simulink model "lato_pc_def"  (Simulink 7.7)
settings: Solver=ode45  StartTime=0.0  StopTime=10.0  RelTol=1e-3
undefined symbols (not defined in the file): DiscIntNeverNeededParam
settings Model: Creator=valeria  LastModifiedBy=valeria

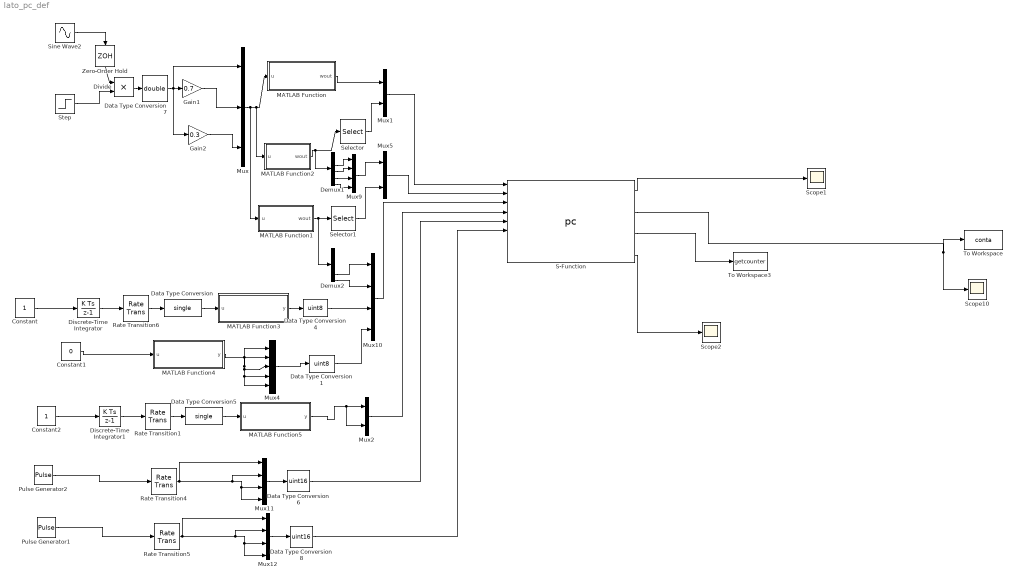
== system lato_pc_def ==
  Constant : Constant  OutDataTypeStr=single
  Constant1 : Constant  Value=0  OutDataTypeStr=single
  Constant2 : Constant  OutDataTypeStr=single
  Data Type Conversion : DataTypeConversion  OutDataTypeStr=single
  Data Type Conversion1 : DataTypeConversion  OutDataTypeStr=uint8
  Data Type Conversion4 : DataTypeConversion  OutDataTypeStr=uint8
  Data Type Conversion5 : DataTypeConversion  OutDataTypeStr=single
  Data Type Conversion6 : DataTypeConversion  OutDataTypeStr=uint16
  Data Type Conversion7 : DataTypeConversion  OutDataTypeStr=double
  Data Type Conversion8 : DataTypeConversion  OutDataTypeStr=uint16
  Demux1 : Demux  Outputs=6
  Demux2 : Demux  Outputs=6
  Discrete-Time Integrator : DiscreteIntegrator  gainval=100  SampleTime=-1  OutDataTypeStr=uint16  ICPrevOutput=DiscIntNeverNeededParam  ICPrevScaledInput=DiscIntNeverNeededParam
  Discrete-Time Integrator1 : DiscreteIntegrator  gainval=100  SampleTime=-1  OutDataTypeStr=uint16  ICPrevOutput=DiscIntNeverNeededParam  ICPrevScaledInput=DiscIntNeverNeededParam
  Divide : Product  Inputs=**
  Gain1 : Gain  Gain=0.7
  Gain2 : Gain  Gain=0.3
  MATLAB Function : Stateflow chart  TreatAsAtomicUnit=on
  MATLAB Function1 : Stateflow chart  TreatAsAtomicUnit=on
  MATLAB Function2 : Stateflow chart  TreatAsAtomicUnit=on
  MATLAB Function3 : Stateflow chart  TreatAsAtomicUnit=on
  MATLAB Function4 : Stateflow chart  TreatAsAtomicUnit=on
  MATLAB Function5 : Stateflow chart  TreatAsAtomicUnit=on
  Mux : Mux  Inputs=3
  Mux1 : Mux  Inputs=2
  Mux{9..12} (4 alike) : Mux
  Mux2 : Mux  Inputs=2
  Mux4 : Mux  Inputs=5
  Mux5 : Mux  Inputs=2
  Pulse Generator1 : DiscretePulseGenerator  PulseType=Time based  Period=10  PulseWidth=5
  Pulse Generator2 : DiscretePulseGenerator  PulseType=Time based  Period=10  PulseWidth=5
  Rate Transition1 : RateTransition
  Rate Transition4 : RateTransition  Deterministic=off
  Rate Transition5 : RateTransition  Deterministic=off
  Rate Transition6 : RateTransition
  S-Function : S-Function  FunctionName=pc  EnableBusSupport=off
  Scope1 : Scope
      settings: YMin=11628  YMax=12852  SaveName=ScopeData2
  Scope10 : Scope
  Scope2 : Scope
      settings: YMin=11628  YMax=12852
  Selector : Selector  InputPortWidth=6  IndexOptions=Index vector (dialog)  Indices=[1 2]  OutputSizes=1
  Selector1 : Selector  InputPortWidth=6  IndexOptions=Index vector (dialog)  Indices=[1 2 3 4]  OutputSizes=1
  Sine Wave2 : Sin  Amplitude=2500*pi/180  SampleTime=0
  Step : Step  SampleTime=0
  To Workspace : ToWorkspace  VariableName=conta  SampleTime=-1  SaveFormat=Structure
  To Workspace3 : ToWorkspace  VariableName=getcounter  SampleTime=-1  SaveFormat=Structure
  Zero-Order Hold : ZeroOrderHold  SampleTime=0.01
  wires:
  S-Function/1 -> Scope1/1
  S-Function/2 -> Scope10/1, To Workspace/1
  S-Function/3 -> To Workspace3/1
  Mux/1 -> MATLAB Function/1(u), MATLAB Function2/1(u), MATLAB Function1/1(u)
  Sine Wave2/1 -> Zero-Order Hold/1
  Data Type Conversion7/1 -> Gain1/1, Mux/1, Gain2/1
  Zero-Order Hold/1 -> Divide/1
  Step/1 -> Divide/2
  Divide/1 -> Data Type Conversion7/1
  Gain2/1 -> Mux/3
  Gain1/1 -> Mux/2
  MATLAB Function2/1(wout) -> Selector/1, Demux1/1
  MATLAB Function/1(wout) -> Mux1/1
  Selector/1 -> Mux1/2
  Mux1/1 -> S-Function/1
  Mux5/1 -> S-Function/2
  MATLAB Function1/1(wout) -> Selector1/1, Demux2/1
  Selector1/1 -> Mux5/2
  Demux1/3 -> Mux9/1
  Demux1/4 -> Mux9/2
  Demux1/5 -> Mux9/3
  Demux1/6 -> Mux9/4
  Mux9/1 -> Mux5/1
  Demux2/5 -> Mux10/1
  Demux2/6 -> Mux10/2
  Mux10/1 -> S-Function/3
  Discrete-Time Integrator/1 -> Rate Transition6/1
  Constant/1 -> Discrete-Time Integrator/1
  Data Type Conversion/1 -> MATLAB Function3/1(u)
  Rate Transition6/1 -> Data Type Conversion/1
  MATLAB Function3/1(y) -> Data Type Conversion4/1
  Constant1/1 -> MATLAB Function4/1(u)
  MATLAB Function4/1(y) -> Mux4/1, Mux4/2, Mux4/3, Mux4/4, Mux4/5
  Mux4/1 -> Data Type Conversion1/1
  Data Type Conversion1/1 -> Mux10/4
  Data Type Conversion4/1 -> Mux10/3
  Discrete-Time Integrator1/1 -> Rate Transition1/1
  Constant2/1 -> Discrete-Time Integrator1/1
  Data Type Conversion5/1 -> MATLAB Function5/1(u)
  Rate Transition1/1 -> Data Type Conversion5/1
  MATLAB Function5/1(y) -> Mux2/1, Mux2/2
  Rate Transition5/1 -> Mux12/1, Mux12/3, Mux12/4, Mux12/2
  Mux12/1 -> Data Type Conversion8/1
  Data Type Conversion8/1 -> S-Function/6
  Pulse Generator1/1 -> Rate Transition5/1
  Rate Transition4/1 -> Mux11/1, Mux11/3, Mux11/4, Mux11/2
  Mux11/1 -> Data Type Conversion6/1
  Pulse Generator2/1 -> Rate Transition4/1
  Data Type Conversion6/1 -> S-Function/5
  Mux2/1 -> S-Function/4
  S-Function/4 -> Scope2/1

== matlab function MATLAB Function1 ==
  data: u input double; wout output double
function wout= magn_fcn(u)
%#codegen

temp = (u(1)*1090);
if temp>(32767), temp=32767; elseif temp<(-32768), temp=-32768; end;
w= comp(temp);
wx_uint8MSB = uint8(bitshift(w, -8));
wx_uint8LSB = uint8(w && uint16(255));

temp = (u(2)*1090);
if temp>(32767), temp=32767; elseif temp<(-32768), temp=-32768; end;
w= comp(temp);
wy_uint8MSB = uint8(bitshift(w, -8));
wy_uint8LSB = uint8(w && uint16(255));


temp = (u(3)*1090);
if temp>(32767), temp=32767; elseif temp<(-32768), temp=-32768; end;
w= comp(temp);
wz_uint8MSB = uint8(bitshift(w, -8));
wz_uint8LSB = uint8(w && uint16(255));

wout = [wx_uint8MSB; wx_uint8LSB; wy_uint8MSB; wy_uint8LSB; wz_uint8MSB; wz_uint8LSB ];
end


function y= comp(u)

%#devo vedere se il numero è positivo o negativo

if(u>0)
   y= uint16(u);  
else
   y= uint16(65536+u);
end
end

== matlab function MATLAB Function ==
  data: u input double; wout output uint8
function wout = gyro_fcn(u)
%#codeg

temp = (u(1)/(0.061*pi/180));
if temp>(32767), temp=32767; elseif temp<(-32768), temp=-32768; end;
w= comp(temp);
wx_uint8MSB = uint8(bitshift(w, -8));
wx_uint8LSB = uint8(w && uint16(255));

temp = (u(2)/(0.061*pi/180));
if temp>(32767), temp=32767; elseif temp<(-32768), temp=-32768; end;
w= comp(temp);
wy_uint8MSB = uint8(bitshift(w, -8));
wy_uint8LSB = uint8(w && uint16(255));


temp = (u(3)/(0.061*pi/180));
if temp>(32767), temp=32767; elseif temp<(-32768), temp=-32768; end;
w= comp(temp);
wz_uint8MSB = uint8(bitshift(w, -8));
wz_uint8LSB = uint8(w && uint16(255));

wout = [wx_uint8MSB; wx_uint8LSB; wy_uint8MSB; wy_uint8LSB; wz_uint8MSB; wz_uint8LSB ];
end


function y= comp(u)

%#devo vedere se il numero è positivo o negativo

if(u>0)
   y= uint16(u);  
else
   y= uint16(65536+u);
end
end

== matlab function MATLAB Function2 ==
  data: u input double; wout output double
function wout = acc_fcn(u)
%#codegen

temp= (u(1)*(256.0*9.81));
if temp>(32767), temp=32767; elseif temp<(-32768), temp=-32768; end;
w= comp(temp);
wx_uint8MSB = uint8(bitshift(w, -8));
wx_uint8LSB = uint8(w && uint16(255));

temp= (u(2)*(256.0*9.81));
if temp>(32767), temp=32767; elseif temp<(-32768), temp=-32768; end;
w= comp(temp);
wy_uint8MSB = uint8(bitshift(w, -8));
wy_uint8LSB = uint8(w && uint16(255));

temp= (u(3)*(256.0*9.81));
if temp>(32767), temp=32767; elseif temp<(-32768), temp=-32768; end;
w= comp(temp);
wz_uint8MSB = uint8(bitshift(w, -8));
wz_uint8LSB = uint8(w && uint16(255));

wout=[wx_uint8MSB; wx_uint8LSB; wy_uint8MSB; wy_uint8LSB; wz_uint8MSB; wz_uint8LSB]; 
end

function y= comp(u)

%#devo vedere se il numero è positivo o negativo

if(u>0)
   y= uint16(u);  
else
   y= uint16(65536+u);
end
end

== matlab function MATLAB Function3 ==
  data: u input single; y output uint32
function y = fcn_single2unit32(u)
%#codegen

y = typecast(u,'uint32');

== matlab function MATLAB Function4 ==
  data: u input single; y output uint32
function y = fcn_single2unit32(u)
%#codegen

y = typecast(u,'uint32');

== matlab function MATLAB Function5 ==
  data: u input single; y output uint32
function y = fcn_single2unit32(u)
%#codegen

y = typecast(u,'uint32');
